simulink model "Pulse_Creator"  (R2014a)
settings: Solver=ode45  StartTime=0.0  StopTime=4  RelTol=1e-3
libraries: simulink x4, powerlib_extras x1
Description:
  | Copyright 2014 The MathWorks, Inc.
settings Model: Creator=smiller  LastModifiedBy=psanghvi
settings DebuggingCC: UnderspecifiedInitializationDetection=Classic  StateNameClashWarn=warning

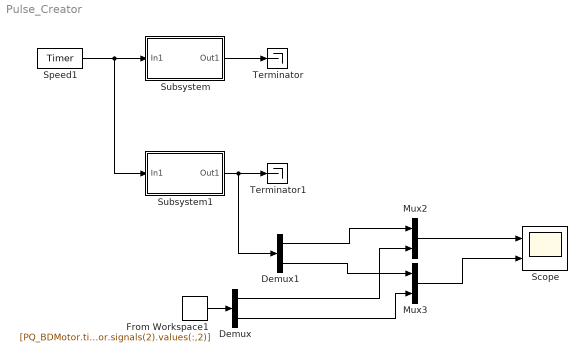
== system Pulse_Creator ==
  Demux : Demux  Outputs=2
  Demux1 : Demux  Outputs=2
  From Workspace1 : FromWorkspace  VariableName=[PQ_BDMotor.time PQ_BDMotor.signals(1).values(:,2) PQ_BDMotor.signals(2).values(:,2)]  SampleTime=0
  Mux2 : Mux  Inputs=2
  Mux3 : Mux  Inputs=2
  Scope : Scope  NumInputPorts=2
      settings: TimeRange=4  YMin=0~-50  YMax=1200~350
  Speed1 : powerlib_extras/Control  Blocks/Timer  t=[0 1.4 1.9 2.4 3]  e=[0 500 0 -500 0]
  Subsystem : Subsystem
  Subsystem1 : Subsystem
  Terminator : Terminator
  Terminator1 : Terminator
  wires:
  Speed1/1 -> Subsystem1/1(In1), Subsystem/1(In1)
  Subsystem/1(Out1) -> Terminator/1
  Subsystem1/1(Out1) -> Demux1/1, Terminator1/1
  From Workspace1/1 -> Demux/1
  Demux1/1 -> Mux2/1
  Demux1/2 -> Mux3/1
  Demux/1 -> Mux2/2
  Mux2/1 -> Scope/1
  Demux/2 -> Mux3/2
  Mux3/1 -> Scope/2

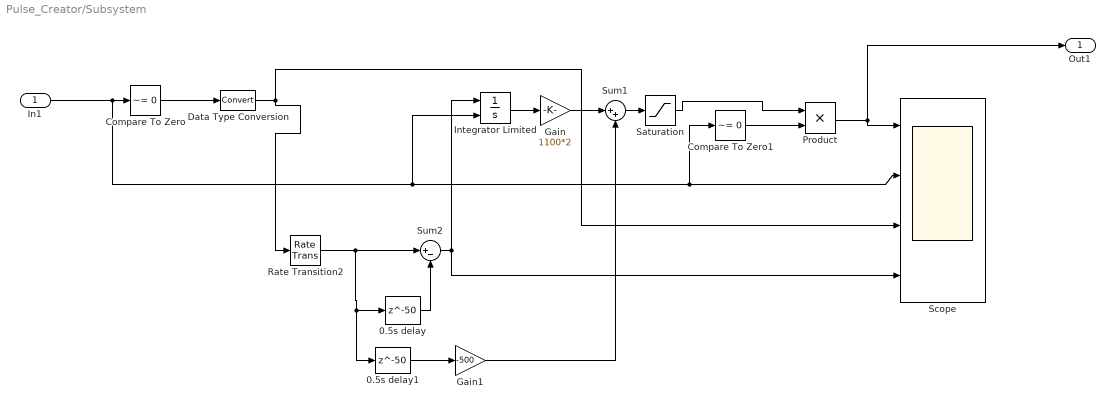
== system Pulse_Creator/Subsystem ==
  In1 : Inport
  0.5s delay : Delay  DelayLength=50  SampleTime=0.01
  0.5s delay1 : Delay  DelayLength=50  SampleTime=0.01
  Compare To Zero : simulink/Logic and Bit Operations/Compare To Zero  relop=~=  OutDataTypeStr=boolean
  Compare To Zero1 : simulink/Logic and Bit Operations/Compare To Zero  relop=~=  OutDataTypeStr=boolean
  Data Type Conversion : DataTypeConversion
  Gain : Gain  Gain=1100*2
  Gain1 : Gain  Gain=-500
  Integrator Limited : Integrator  ExternalReset=falling  LimitOutput=on  UpperSaturationLimit=1  LowerSaturationLimit=0
  Product : Product
  Rate Transition2 : RateTransition  OutPortSampleTime=0.01
  Saturation : Saturate  UpperLimit=1100  LowerLimit=0
  Scope : Scope  NumInputPorts=4
      settings: TimeRange=10  YMin=0~-1~0~-1  YMax=2000~1~1~1
  Sum1 : Sum  Inputs=|++  SaturateOnIntegerOverflow=on  InputSameDT=on  OutDataTypeStr=Inherit: Same as first input
  Sum2 : Sum  Inputs=|+-  SaturateOnIntegerOverflow=on  InputSameDT=on  OutDataTypeStr=Inherit: Same as first input
  Out1 : Outport
  wires:
  Compare To Zero/1 -> Data Type Conversion/1
  In1/1 -> Compare To Zero/1, Compare To Zero1/1, Scope/2, Integrator Limited/2
  Integrator Limited/1 -> Gain/1
  Data Type Conversion/1 -> Scope/3, Rate Transition2/1
  Gain/1 -> Sum1/1
  0.5s delay/1 -> Sum2/2
  Rate Transition2/1 -> Sum2/1, 0.5s delay1/1, 0.5s delay/1
  Sum2/1 -> Integrator Limited/1, Scope/4
  Product/1 -> Out1/1, Scope/1
  Gain1/1 -> Sum1/2
  0.5s delay1/1 -> Gain1/1
  Sum1/1 -> Saturation/1
  Saturation/1 -> Product/1
  Compare To Zero1/1 -> Product/2

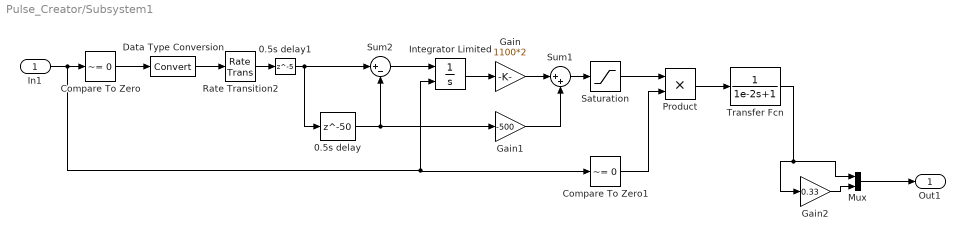
== system Pulse_Creator/Subsystem1 ==
  In1 : Inport
  0.5s delay : Delay  DelayLength=50  SampleTime=0.01
  0.5s delay1 : Delay  DelayLength=5  SampleTime=0.01
  Compare To Zero : simulink/Logic and Bit Operations/Compare To Zero  relop=~=  OutDataTypeStr=boolean
  Compare To Zero1 : simulink/Logic and Bit Operations/Compare To Zero  relop=~=  OutDataTypeStr=boolean
  Data Type Conversion : DataTypeConversion
  Gain : Gain  Gain=1100*2
  Gain1 : Gain  Gain=-500
  Gain2 : Gain  Gain=0.33
  Integrator Limited : Integrator  ExternalReset=falling  LimitOutput=on  UpperSaturationLimit=1  LowerSaturationLimit=0
  Mux : Mux  Inputs=2
  Product : Product
  Rate Transition2 : RateTransition  OutPortSampleTime=0.01
  Saturation : Saturate  UpperLimit=1100  LowerLimit=0
  Sum1 : Sum  Inputs=|++  SaturateOnIntegerOverflow=on  InputSameDT=on  OutDataTypeStr=Inherit: Same as first input
  Sum2 : Sum  Inputs=|+-  SaturateOnIntegerOverflow=on  InputSameDT=on  OutDataTypeStr=Inherit: Same as first input
  Transfer Fcn : TransferFcn  Denominator=[1e-2 1]
  Out1 : Outport
  wires:
  Compare To Zero1/1 -> Product/2
  Saturation/1 -> Product/1
  Sum1/1 -> Saturation/1
  0.5s delay/1 -> Sum2/2, Gain1/1
  Gain1/1 -> Sum1/2
  Product/1 -> Transfer Fcn/1
  Sum2/1 -> Integrator Limited/1
  Rate Transition2/1 -> 0.5s delay1/1
  Gain/1 -> Sum1/1
  Data Type Conversion/1 -> Rate Transition2/1
  Integrator Limited/1 -> Gain/1
  In1/1 -> Integrator Limited/2, Compare To Zero1/1, Compare To Zero/1
  Compare To Zero/1 -> Data Type Conversion/1
  Transfer Fcn/1 -> Mux/1, Gain2/1
  Gain2/1 -> Mux/2
  Mux/1 -> Out1/1
  0.5s delay1/1 -> 0.5s delay/1, Sum2/1
